simulink library "WECSim_Lib"  (R2014b)
settings: Solver=ode45  StartTime=0.0  StopTime=10.0  RelTol=1e-3
undefined symbols (not defined in the file): body, constraint, pto, simu, waves, X, Y, Z
libraries: nesl_utility x178, sm_lib x59, vrlib x12
(part 4 of 6)

== system WECSim_Lib/Body Elements/Rigid Body/Structure ==
  note: SimMechanics Model
      |
      | Body: Consists of body properties (inertia and vizualisation) defined at the CG, and a connection point at (0,0,0), the free surface.
      |
      | Forces::  Total forces calculated by WEC-Sim are applied at the Body CG. Other forces (constraints and PTOs) can be applied outside of this block, though the connection point.
      |
      | Motion Sensor: Measures the displacement, velocity, and acceleration of the Body CG relative to the world frame.
  note: body.mass
      | body.momOfInertia
      | body.geometryFile (set through Rigid Body mask)
      | body.hydroData.properties.cg
      | body.initDisp.initAngularDispAxis
      | body.initDisp.initAngularDispAngle
      | body.initDisp.initLinDisp
  Total Force : Inport
  Body Properties : sm_lib/Body Elements/Solid  InertiaType=Custom  Mass=body.mass  MassUnits=kg  CenterOfMass=[0 0 0]  CenterOfMassUnits=m  MomentsOfInertia=body.momOfInertia  MomentsOfInertiaUnits=kg*m^2  ProductsOfInertia=[0 0 0]  ProductsOfInertiaUnits=kg*m^2  DensityBased=on  Density=1000  DensityUnits=kg/(m^3)  GraphicType=FromGeometry  MarkerShape=Sphere  MarkerSize=10  MarkerSizeUnits=m  GraphicVisPropType=SimpleVisualProperties  GraphicDiffuseColor=body.viz.color  GraphicSpecularColor=[0.5 0.5 0.5 1.0]  GraphicAmbientColor=[0.15 0.15 0.15 1.0]  GraphicEmissiveColor=[0.0 0.0 0.0 1.0]  GraphicShininess=75  GraphicOpacity=body.viz.opacity  GeometryShape=FromFile  RectangleSize=[1 1]  RectangleSizeUnits=m  BrickDimensions=[1 1 1]  BrickDimensionUnits=m  CylinderRadius=1  CylinderRadiusUnits=m  CylinderLength=1  CylinderLengthUnits=m  SphereRadius=1  SphereRadiusUnits=m  EllipsoidRadii=[1 1 1]  EllipsoidRadiiUnits=m  ExtrusionCrossSection=[1 1; -1 1; -1 -1; 1 -1]  ExtrusionCrossSectionUnits=m  ExtrusionLength=1  ExtrusionLengthUnits=m  PolygonNumSides=3  PolygonOuterRadius=1  PolygonOuterRadiusUnits=m  ExtGeomFileType=STL  ExtGeomFileName=geometry/float.stl  ExtGeomFileUnits=m  RevolutionCrossSection=[1 1; 1 -1; 2 -1; 2 1]  RevolutionCrossSectionUnits=m  RevolutionExtent=Full  RevolutionAngle=180  RevolutionAngleUnits=deg  BlockFunction=simmechanics.library.body_elements.solid
  External Force and Torque : sm_lib/Forces and Torques/External Force and Torque  ForceResolutionFrame=World  EnableForceX=off  EnableForceY=off  EnableForceZ=off  EnableForce=on  TorqueResolutionFrame=World  EnableTorqueX=off  EnableTorqueY=off  EnableTorqueZ=off  EnableTorque=on  BlockFunction=simmechanics.library.forces_torques.external_force_torque
  Motion Sensor : Subsystem
  Rigid Transform (Setup CG) : sm_lib/Frames and Transforms/Rigid Transform  TranslationMethod=Cartesian  TranslationLengthUnit=m  TranslationStandardAxis=+Z  TranslationStandardOffset=0  TranslationCartesianOffset=body.hydroData.properties.cg  TranslationROffset=0  TranslationROffsetUnits=m  TranslationZOffset=0  TranslationZOffsetUnits=m  TranslationThetaOffset=0  TranslationThetaOffsetUnits=deg  RotationMethod=None  RotationAngleUnits=rad  RotationStandardAxis=+Y  RotationAngle=0.05  RotationArbitraryAxis=[0.57735026918962584 0.57735026918962584 0.57735026918962584]  FollAlignAxisA=+X  BaseAlignAxisA=+Y  FollAlignAxisB=+Y  BaseAlignAxisB=+Z  RotationMatrix=[1 0 0; 0 1 0; 0 0 1]  BlockFunction=simmechanics.library.frames_transforms.rigid_transform
  Rigid Transform (Setup Initial Disp) : sm_lib/Frames and Transforms/Rigid Transform  TranslationMethod=Cartesian  TranslationLengthUnit=m  TranslationStandardAxis=+Z  TranslationStandardOffset=0  TranslationCartesianOffset=body.initDisp.initLinDisp  TranslationROffset=0  TranslationROffsetUnits=m  TranslationZOffset=0  TranslationZOffsetUnits=m  TranslationThetaOffset=0  TranslationThetaOffsetUnits=deg  RotationMethod=ArbitraryAxis  RotationAngleUnits=rad  RotationStandardAxis=+Y  RotationAngle=body.initDisp.initAngularDispAngle  RotationArbitraryAxis=body.initDisp.initAngularDispAxis  FollAlignAxisA=+X  BaseAlignAxisA=+Y  FollAlignAxisB=+Y  BaseAlignAxisB=+Z  RotationMatrix=[1 0 0; 0 1 0; 0 0 1]  BlockFunction=simmechanics.library.frames_transforms.rigid_transform
  Selector : Selector  InputPortWidth=6  Indices=[1:3]
  Selector1 : Selector  InputPortWidth=6  Indices=[4:6]
  Simulink-PS Converter1 : nesl_utility/Simulink-PS Converter  PhysicalDomain=network_engine_domain  SubClassName=ps_input  LeftPortType=input  RightPortType=output  PseudoPeriodic=off  Frequencies=[]  NoiseDistribution=none  NoiseParameters=[]  Unit=1  AffineConversion=off  InputFiltering=off  SimscapeFilterOrder=1  InputFilterTimeConstant=0.001  UdotUserProvided=1
  Simulink-PS Converter2 : nesl_utility/Simulink-PS Converter  PhysicalDomain=network_engine_domain  SubClassName=ps_input  LeftPortType=input  RightPortType=output  PseudoPeriodic=off  Frequencies=[]  NoiseDistribution=none  NoiseParameters=[]  Unit=1  AffineConversion=off  InputFiltering=off  SimscapeFilterOrder=1  InputFilterTimeConstant=0.001  UdotUserProvided=1
  World Frame : sm_lib/Frames and Transforms/World Frame  BlockFunction=simmechanics.library.frames_transforms.world_frame
  Conn Free Surface : PMIOPort  Port=1  Side=Right
  Response : Outport
  wires:
  Motion Sensor/1(Response) -> Response/1
  Selector1/1 -> Simulink-PS Converter2/1
  Selector/1 -> Simulink-PS Converter1/1
  Total Force/1 -> Selector/1, Selector1/1
  connections:
  World Frame/RConn1 -- Motion Sensor/LConn1
  Rigid Transform (Setup Initial Disp)/LConn1 -- Rigid Transform (Setup CG)/RConn1
  Conn Free Surface/RConn1 -- Rigid Transform (Setup CG)/LConn1
  Motion Sensor/RConn1 -- External Force and Torque/RConn1 -- Body Properties/RConn1 -- Rigid Transform (Setup Initial Disp)/RConn1
  External Force and Torque/LConn2 -- Simulink-PS Converter2/RConn1
  External Force and Torque/LConn1 -- Simulink-PS Converter1/RConn1

== system WECSim_Lib/Body Elements/Rigid Body/Wave Diffraction and Excitation Force Calculation ==
  note: Calculates the excitation force, F_Excitation, given by
      | F_Excitation = R * F_wave.
      |
      | There are two cases for Calculating the Ramp function, R:
      |    1. simulation Time is less than Ramp Time: Apply ramp function
      |    2. Simulation time is larger than Ramp Time: Do not apply ramp function (R=1)
      |
      | Similarly there are two cases for the wave force, F_wave: Regular and Irregular waves.
      |
      | Notes:
      | Output dimension set to '6' in output port to eliminate singleton dimension.
  Time : Inport
  Displacement : Inport  Port=2
  WaveElv : Inport  Port=3
  Add : Sum
  If2 : If  NumInputs=2  IfExpression=u1 < u2
  Linear Wave Excitation Force Variant Subsystem : Subsystem  Variant=on
  Merge1 : Merge
  No Ramp Function : Subsystem  TreatAsAtomicUnit=on
  Nonlinear FK Force Variant Subsystem : Subsystem  Variant=on
  Product : Product
  Ramp Function : Subsystem  TreatAsAtomicUnit=on
  Ramp Function Time1 : Constant  Value=simu.rampT
  F_Excitation : Outport  PortDimensions=6
  wires:
  No Ramp Function/1(R) -> Merge1/2
  Ramp Function/1(R) -> Merge1/1
  If2/1 -> Ramp Function/Action
  If2/2 -> No Ramp Function/Action
  Ramp Function Time1/1 -> If2/2
  Merge1/1 -> Product/1  "R"
  Time/1 -> Linear Wave Excitation Force Variant Subsystem/1(In1), Nonlinear FK Force Variant Subsystem/1(In1), Ramp Function/1(Time), If2/1
  Add/1 -> Product/2  "F_wave"
  Product/1 -> F_Excitation/1  "F_Excitation"
  Displacement/1 -> Nonlinear FK Force Variant Subsystem/2(In2)
  WaveElv/1 -> Nonlinear FK Force Variant Subsystem/3(In3)
  Linear Wave Excitation Force Variant Subsystem/1(Out1) -> Add/1
  Nonlinear FK Force Variant Subsystem/1(Out1) -> Add/2

== system WECSim_Lib/Body Elements/Rigid Body/Wave Radiation Forces Calculation ==
  note: Calculates the wave radiation forces:
      | 	Added Mass Force = added mass matrix * acceleration vector
      | 	Single frequency radiation damping force = radiation damping matrix * acceleration vector
      | 	Convolution Integral
      |
      | The code can run in one of two modes:
      | 	Convolution integral: the radiation damping matrix is set to zero, and the infinite frequency added mass is used.
      | 	Single Frequency: The impulse response function K is set to zero, and the radiation damping and added mass matrices for the specified frequency are used.
      |
      | This is set by the body.hydroForcePre method, based on the specified wave type.
  Velocity : Inport
  Acceleration : Inport  Port=2
  Time : Inport  Port=3
  Added Mass Matrix : Constant  Value=body.hydroForce.fAddedMass
  Product1 : Product  Multiplication=Matrix(*)
  SS CI and Constant-Damping-CoeVariant Subsystem : Subsystem  Variant=on
  Transport Delay : TransportDelay  DelayTime=10e-8
  F_RadiationDamping : Outport
  F_AddedMass : Outport  Port=2
  wires:
  Added Mass Matrix/1 -> Product1/1
  Product1/1 -> F_AddedMass/1  "F_AddedMass"
  Velocity/1 -> SS CI and Constant-Damping-CoeVariant Subsystem/1(In1)
  SS CI and Constant-Damping-CoeVariant Subsystem/1(Out1) -> F_RadiationDamping/1  "F_RadiationDamping"
  Transport Delay/1 -> Product1/2
  Acceleration/1 -> Transport Delay/1
  Time/1 -> SS CI and Constant-Damping-CoeVariant Subsystem/2(In2)

== system WECSim_Lib/Constraints/Floating (3DOF)/Mooring ==
  note: 1) Add Subsystem or Model blocks as valid variant choices.
      | 2) You cannot connect blocks at this level. At simulation, connectivity is automatically
      | determined, based on the active variant and port name matching.
  Displacement : Inport
  Clock : Inport  Port=2
  Velocity : Inport  Port=3
  MoorDyn : Subsystem  VariantControl=sv_moorDyn
  Mooring Matrix : Subsystem  VariantControl=sv_mooringMatrix
  F_Mooring : Outport

== system WECSim_Lib/Constraints/Floating (6DOF)/Mooring ==
  note: 1) Add Subsystem or Model blocks as valid variant choices.
      | 2) You cannot connect blocks at this level. At simulation, connectivity is automatically
      | determined, based on the active variant and port name matching.
  Displacement : Inport
  Clock : Inport  Port=2
  Velocity : Inport  Port=3
  MoorDyn : Subsystem  VariantControl=sv_moorDyn
  Mooring Matrix : Subsystem  VariantControl=sv_mooringMatrix
  F_Mooring : Outport

== system WECSim_Lib/Constraints/Heave/Mooring ==
  note: 1) Add Subsystem or Model blocks as valid variant choices.
      | 2) You cannot connect blocks at this level. At simulation, connectivity is automatically
      | determined, based on the active variant and port name matching.
  Displacement : Inport
  Clock : Inport  Port=2
  Velocity : Inport  Port=3
  MoorDyn : Subsystem  VariantControl=sv_moorDyn
  Mooring Matrix : Subsystem  VariantControl=sv_mooringMatrix
  F_Mooring : Outport

== system WECSim_Lib/Constraints/Pitch/Mooring ==
  note: 1) Add Subsystem or Model blocks as valid variant choices.
      | 2) You cannot connect blocks at this level. At simulation, connectivity is automatically
      | determined, based on the active variant and port name matching.
  Displacement : Inport
  Clock : Inport  Port=2
  Velocity : Inport  Port=3
  MoorDyn : Subsystem  VariantControl=sv_moorDyn
  Mooring Matrix : Subsystem  VariantControl=sv_mooringMatrix
  F_Mooring : Outport

== system WECSim_Lib/Constraints/Surge/Mooring ==
  note: 1) Add Subsystem or Model blocks as valid variant choices.
      | 2) You cannot connect blocks at this level. At simulation, connectivity is automatically
      | determined, based on the active variant and port name matching.
  Displacement : Inport
  Clock : Inport  Port=2
  Velocity : Inport  Port=3
  MoorDyn : Subsystem  VariantControl=sv_moorDyn
  Mooring Matrix : Subsystem  VariantControl=sv_mooringMatrix
  F_Mooring : Outport

== system WECSim_Lib/PTOs/Rotational PTO (Local RY)/InternalMechanics ==
  note: Calculate PTO force and power.
      |
      | F_pto  = k*x + c*v,
      | where F_pto is the force the PTO applies to the body (at the PTO location), x and v are the joint position and velocity.
      |
      | The power extracted is
      | P = c * v^2
  Position : Inport
  Velocity : Inport  Port=2
  Add : Sum  Inputs=--
  Math Function : Math  Operator=square  SaturateOnIntegerOverflow=on
  PCC Damping Coefficient : Constant  Value=pto.c
  PCC Stiffness Coefficient : Constant  Value=pto.k
  Product : Product  Inputs=**
  Product1 : Product  Inputs=**
  Product2 : Product  Inputs=**
  Force : Outport
  Power : Outport  Port=2
  wires:
  PCC Damping Coefficient/1 -> Product2/1, Product1/1
  Product2/1 -> Power/1
  Velocity/1 -> Math Function/1, Product1/2
  PCC Stiffness Coefficient/1 -> Product/2
  Position/1 -> Product/1
  Add/1 -> Force/1
  Math Function/1 -> Product2/2
  Product/1 -> Add/1
  Product1/1 -> Add/2

== system WECSim_Lib/PTOs/Rotational PTO Prescribed Motion (Local RY)/InternalMechanics ==
  note: Calculate PTO force and power.
      |
      | F_pto  = k*x + c*v,
      | where F_pto is the force the PTO applies to the body (at the PTO location), x and v are the joint position and velocity.
      |
      | The power extracted is
      | P = c * v^2
  Position : Inport
  Velocity : Inport  Port=2
  Add : Sum  Inputs=--
  Math Function : Math  Operator=square  SaturateOnIntegerOverflow=on
  PCC Damping Coefficient : Constant  Value=pto.c
  PCC Stiffness Coefficient : Constant  Value=pto.k
  Product : Product  Inputs=**
  Product1 : Product  Inputs=**
  Product2 : Product  Inputs=**
  Force : Outport
  Power : Outport  Port=2
  wires:
  PCC Damping Coefficient/1 -> Product2/1, Product1/1
  Product2/1 -> Power/1
  Velocity/1 -> Math Function/1, Product1/2
  PCC Stiffness Coefficient/1 -> Product/2
  Position/1 -> Product/1
  Add/1 -> Force/1
  Math Function/1 -> Product2/2
  Product/1 -> Add/1
  Product1/1 -> Add/2

== system WECSim_Lib/PTOs/Rotational PTO UD Torque (Local RY)/InternalMechanics ==
  note: Calculate PTO force and power.
      |
      | F_pto  = k*x + c*v,
      | where F_pto is the force the PTO applies to the body (at the PTO location), x and v are the joint position and velocity.
      |
      | The power extracted is
      | P = c * v^2
  Position : Inport
  Velocity : Inport  Port=2
  Add : Sum  Inputs=--
  Math Function : Math  Operator=square  SaturateOnIntegerOverflow=on
  PCC Damping Coefficient : Constant  Value=pto.c
  PCC Stiffness Coefficient : Constant  Value=pto.k
  Product : Product  Inputs=**
  Product1 : Product  Inputs=**
  Product2 : Product  Inputs=**
  Force : Outport
  Power : Outport  Port=2
  wires:
  Product1/1 -> Add/2
  Product/1 -> Add/1
  Math Function/1 -> Product2/2
  Add/1 -> Force/1
  Position/1 -> Product/1
  PCC Stiffness Coefficient/1 -> Product/2
  Velocity/1 -> Product1/2, Math Function/1
  Product2/1 -> Power/1
  PCC Damping Coefficient/1 -> Product1/1, Product2/1

== system WECSim_Lib/PTOs/Translational PTO (Local X)/ForceAndPower ==
  note: Calculate PTO force and power.
      |
      | F_pto  = k*x + c*v,
      | where F_pto is the force the PTO applies to the body (at the PTO location), x and v are the joint position and velocity.
      |
      | The power extracted is
      | P = c * v^2
  Pos : Inport
  Vel : Inport  Port=2
  Add : Sum  Inputs=--
  Math Function : Math  Operator=square  SaturateOnIntegerOverflow=on
  PCC Damping Coefficient : Constant  Value=pto.c
  PCC Stiffness Coefficient : Constant  Value=pto.k
  Product : Product  Inputs=**
  Product1 : Product  Inputs=**
  Product2 : Product  Inputs=**
  Force : Outport
  Power : Outport  Port=2
  wires:
  PCC Damping Coefficient/1 -> Product1/1, Product2/1
  Product2/1 -> Power/1
  Vel/1 -> Product1/2, Math Function/1
  PCC Stiffness Coefficient/1 -> Product/2
  Pos/1 -> Product/1
  Add/1 -> Force/1
  Math Function/1 -> Product2/2
  Product/1 -> Add/1
  Product1/1 -> Add/2

== system WECSim_Lib/PTOs/Translational PTO (Local Z)/InternalMechanics ==
  note: Calculate PTO force and power.
      |
      | F_pto  = k*x + c*v,
      | where F_pto is the force the PTO applies to the body (at the PTO location), x and v are the joint position and velocity.
      |
      | The power extracted is
      | P = c * v^2
  Position : Inport
  Velocity : Inport  Port=2
  Add : Sum  Inputs=--
  Math Function : Math  Operator=square  SaturateOnIntegerOverflow=on
  PCC Damping Coefficient : Constant  Value=pto.c
  PCC Stiffness Coefficient : Constant  Value=pto.k
  Product : Product  Inputs=**
  Product1 : Product  Inputs=**
  Product2 : Product  Inputs=**
  Force : Outport
  Power : Outport  Port=2
  wires:
  PCC Damping Coefficient/1 -> Product2/1, Product1/1
  Product2/1 -> Power/1
  Velocity/1 -> Math Function/1, Product1/2
  PCC Stiffness Coefficient/1 -> Product/2
  Position/1 -> Product/1
  Add/1 -> Force/1
  Math Function/1 -> Product2/2
  Product/1 -> Add/1
  Product1/1 -> Add/2

== system WECSim_Lib/PTOs/Translational PTO Prescribed Motion (Local X)/ForceAndPower ==
  note: Calculate PTO force and power.
      |
      | F_pto  = k*x + c*v,
      | where F_pto is the force the PTO applies to the body (at the PTO location), x and v are the joint position and velocity.
      |
      | The power extracted is
      | P = c * v^2
  Pos : Inport
  Vel : Inport  Port=2
  Add : Sum  Inputs=--
  Math Function : Math  Operator=square  SaturateOnIntegerOverflow=on
  PCC Damping Coefficient : Constant  Value=pto.c
  PCC Stiffness Coefficient : Constant  Value=pto.k
  Product : Product  Inputs=**
  Product1 : Product  Inputs=**
  Product2 : Product  Inputs=**
  Force : Outport
  Power : Outport  Port=2
  wires:
  Product1/1 -> Add/2
  Product/1 -> Add/1
  Math Function/1 -> Product2/2
  Add/1 -> Force/1
  Pos/1 -> Product/1
  PCC Stiffness Coefficient/1 -> Product/2
  Vel/1 -> Math Function/1, Product1/2
  Product2/1 -> Power/1
  PCC Damping Coefficient/1 -> Product2/1, Product1/1

== system WECSim_Lib/PTOs/Translational PTO Prescribed Motion (Local Z)/InternalMechanics ==
  note: Calculate PTO force and power.
      |
      | F_pto  = k*x + c*v,
      | where F_pto is the force the PTO applies to the body (at the PTO location), x and v are the joint position and velocity.
      |
      | The power extracted is
      | P = c * v^2
  Position : Inport
  Velocity : Inport  Port=2
  Add : Sum  Inputs=--
  Math Function : Math  Operator=square  SaturateOnIntegerOverflow=on
  PCC Damping Coefficient : Constant  Value=pto.c
  PCC Stiffness Coefficient : Constant  Value=pto.k
  Product : Product  Inputs=**
  Product1 : Product  Inputs=**
  Product2 : Product  Inputs=**
  Force : Outport
  Power : Outport  Port=2
  wires:
  PCC Damping Coefficient/1 -> Product2/1, Product1/1
  Product2/1 -> Power/1
  Velocity/1 -> Math Function/1, Product1/2
  PCC Stiffness Coefficient/1 -> Product/2
  Position/1 -> Product/1
  Add/1 -> Force/1
  Math Function/1 -> Product2/2
  Product/1 -> Add/1
  Product1/1 -> Add/2

== system WECSim_Lib/PTOs/Translational PTO UD Force (Local X)/ForceAndPower ==
  note: Calculate PTO force and power.
      |
      | F_pto  = k*x + c*v,
      | where F_pto is the force the PTO applies to the body (at the PTO location), x and v are the joint position and velocity.
      |
      | The power extracted is
      | P = c * v^2
  Pos : Inport
  Vel : Inport  Port=2
  Add : Sum  Inputs=--
  Math Function : Math  Operator=square  SaturateOnIntegerOverflow=on
  PCC Damping Coefficient : Constant  Value=pto.c
  PCC Stiffness Coefficient : Constant  Value=pto.k
  Product : Product  Inputs=**
  Product1 : Product  Inputs=**
  Product2 : Product  Inputs=**
  Force : Outport
  Power : Outport  Port=2
  wires:
  PCC Damping Coefficient/1 -> Product1/1, Product2/1
  Product2/1 -> Power/1
  Vel/1 -> Product1/2, Math Function/1
  PCC Stiffness Coefficient/1 -> Product/2
  Pos/1 -> Product/1
  Add/1 -> Force/1
  Math Function/1 -> Product2/2
  Product/1 -> Add/1
  Product1/1 -> Add/2

== system WECSim_Lib/PTOs/Translational PTO UD Force (Local Z)/InternalMechanics ==
  note: Calculate PTO force and power.
      |
      | F_pto  = k*x + c*v,
      | where F_pto is the force the PTO applies to the body (at the PTO location), x and v are the joint position and velocity.
      |
      | The power extracted is
      | P = c * v^2
  Position : Inport
  Velocity : Inport  Port=2
  Add : Sum  Inputs=--
  Math Function : Math  Operator=square  SaturateOnIntegerOverflow=on
  PCC Damping Coefficient : Constant  Value=pto.c
  PCC Stiffness Coefficient : Constant  Value=pto.k
  Product : Product  Inputs=**
  Product1 : Product  Inputs=**
  Product2 : Product  Inputs=**
  Force : Outport
  Power : Outport  Port=2
  wires:
  Product1/1 -> Add/2
  Product/1 -> Add/1
  Math Function/1 -> Product2/2
  Add/1 -> Force/1
  Position/1 -> Product/1
  PCC Stiffness Coefficient/1 -> Product/2
  Velocity/1 -> Product1/2, Math Function/1
  Product2/1 -> Power/1
  PCC Damping Coefficient/1 -> Product1/1, Product2/1

== system WECSim_Lib/Body Elements/Rigid Body/B2B Subsystem/B2B ==
  CrossCoupling : Subsystem  mask{body=body}
      mask prompts: body "Body Number"
      mask help: This is used to
      mask init:
      | %In the initialization tab we place the code modifying the block
      | 
      | cb = gcb;
      | % position of initial blocks
      | set_param([cb '/vel1'],'Position',[200 1*50 240 (1*50+30)])
      | set_param([cb '/BC1'], 'Position',[375 40 380 90])
      | set_param([cb '/vel'], 'Position',[410 59 440 71])
      | set_param([cb '/acc1'],'Position',[600 1*50 640 (1*50+30)])
      | set_param([cb '/BC2'], 'Position',[775 40 780 90])
      | set_param([cb '/acc'], 'Position',[810 59 840 71])
      | 
      | % add/delete lines & blocks
      | newInputs = 0;
      | numbodies = body.bodyTotal;
      | iBod = 2;
      | while iBod < 100
      |     try 
      |         find_system([cb,'/vel',num2str(iBod)],'Type','Block');
      |         if iBod > numbodies
      |             %delete 'From' blocks and lines if bodynumber > total bodies
      |             delete_line(cb,['vel',num2str(iBod),'/1'],['BC',num2str(1),'/',num2str(iBod)])
      |             delete_line(cb,['acc',num2str(iBod),'/1'],['BC',num2str(2),'/',num2str(iBod)])
      |             delete_block([cb '/vel',num2str(iBod)])
      |             delete_block([cb '/acc',num2str(iBod)])
      |         end
      |     catch
      |         %set number of outputs for 'Bus Creator' blocks 
      |         if newInputs==0
      |             set_param([cb,'/BC1'],'Inputs',num2str(numbodies))
      |             set_param([cb,'/BC2'],'Inputs',num2str(numbodies))
      |         end
      |         if iBod <= numbodies
      |             newInputs = newInputs + 1;
      |             %add velocity 'From' block
      |             add_block('simulink/Signal Routing/From', [cb,'/vel',num2str(iBod)],'MakeNameUnique', 'on',...
      |             'Position',[200 iBod*50 240 (iBod*50+30)], 'BackgroundColor','green')
      |             h=[cb,'/vel',num2str(iBod)];
      |             responseName=['vel' num2str(iBod)];
      |             set_param(h,'GotoTag',responseName);
      |             %add acceleration 'From' block
      |             add_block('simulink/Signal Routing/From', [cb,'/acc',num2str(iBod)],'MakeNameUnique', 'on',...
      |             'Position',[600 iBod*50 640 (iBod*50+30)], 'BackgroundColor','green')
      |             h=[cb,'/acc',num2str(iBod)];
      |             responseName=['acc' num2str(iBod)];
      |             set_param(h,'GotoTag',responseName);
      |             %add lines
      |             add_line(cb,['vel',num2str(iBod),'/1'],['BC',num2str(1),'/',num2str(iBod)])
      |             add_line(cb,['acc',num2str(iBod),'/1'],['BC',num2str(2),'/',num2str(iBod)])
      |         else
      |             break
      |         end
      |     end
      |     iBod = iBod + 1;
      | end
      mask Callback body: %customsat_callback('input',gcb)
      mask DialogControl DescTextVar Prompt: This block transfers the velocity and acceleration vectors between bodies allowing for the coupled hydrodynamic forces to be calculated.  This block should not be included if there is only one body or if the hydrodynamic coupling parameter is set to 'No' in the rigid body block.
  vel : Outport
  acc : Outport  Port=2
  wires:
  CrossCoupling/1(vel) -> vel/1
  CrossCoupling/2(acc) -> acc/1

== system WECSim_Lib/Body Elements/Rigid Body/B2B Subsystem/noB2B ==
  vel_in : Inport
  acc_in : Inport  Port=2
  vel : Outport
  acc : Outport  Port=2
  wires:
  vel_in/1 -> vel/1  "x"
  acc_in/1 -> acc/1

== system WECSim_Lib/Body Elements/Rigid Body/Hydrostatic Restoring Force Calculation/Linear and Nonlinear Restoring Force Variant Subsystem ==
  note: 1) Add Subsystem or Model blocks as valid variant choices.
      | 2) You cannot connect blocks at this level. At simulation, connectivity is automatically
      | determined, based on the active variant and port name matching.
  In1 : Inport
  In2 : Inport  Port=2
  In3 : Inport  Port=3
  "Linear Hydrostatic Restoring Force " : Subsystem  VariantControl=sv_linearHydro
  Nonlinear Hydrostatic Restoring Force : Subsystem  VariantControl=sv_nonlinearHydro
  Out1 : Outport

== system WECSim_Lib/Body Elements/Rigid Body/Morrison Element and ViscousDampingForceCalculation/Morrison Element Variant Subsystem ==
  note: 1) Add Subsystem or Model blocks as valid variant choices.
      | 2) You cannot connect blocks at this level. At simulation, connectivity is automatically
      | determined, based on the active variant and port name matching.
  In1 : Inport
  In2 : Inport  Port=2
  In3 : Inport  Port=3
  Morrison Element Off : Subsystem  VariantControl=sv_MEOff
  Morrison Element On : Subsystem  Variant=on  VariantControl=sv_MEOn
  Out1 : Outport

== system WECSim_Lib/Body Elements/Rigid Body/Nonlinear Wave Elevation/Linear or Instantaneous Free Surface ==
  note: 1) Add Subsystem or Model blocks as valid variant choices.
      | 2) You cannot connect blocks at this level. At simulation, connectivity is automatically
      | determined, based on the active variant and port name matching.
  In1 : Inport
  In2 : Inport  Port=2
  "Instantaneous Water Free Surface  " : Subsystem  VariantControl=sv_instFS
  "Mean Water Free Surface " : Subsystem  VariantControl=sv_meanFS
  Out1 : Outport

== system WECSim_Lib/Body Elements/Rigid Body/Structure/Motion Sensor ==
  note: Measures the position, velocity, and acceleration of the follower (F) frame relative to the base (B) frame.
      | Ouputs a bus of 3 signals, each signal is a vector length 6.
  Angle : MATLAB Function  TreatAsAtomicUnit=on
  Bus Creator : BusCreator  Inputs=3
  Mux : Mux
  Mux1 : Mux  Inputs=6
  Mux2 : Mux  Inputs=6
  PS-Simulink Converter{,1..15} (16 alike) : nesl_utility/PS-Simulink Converter  PhysicalDomain=network_engine_domain  SubClassName=ps_output  LeftPortType=input  RightPortType=output  PseudoPeriodic=off  Frequencies=[]  Unit=1  AffineConversion=off
  Transform Sensor : sm_lib/Frames and Transforms/Transform Sensor  MeasurementFrame=World  SenseAngle=off  SenseAxis=off  SenseAngle1=off  SenseAngle2=off  SenseAngle3=off  SenseQ=on  SenseR=off  SenseOmegaX=on  SenseOmegaY=on  SenseOmegaZ=on  SenseOmega1=off  SenseOmega2=off  SenseOmega3=off  SenseQDot=off  SenseRDot=off  SenseAlphaX=on  SenseAlphaY=on  SenseAlphaZ=on  SenseAlpha1=off  SenseAlpha2=off  SenseAlpha3=off  SenseQDDot=off  SenseRDDot=off  SenseX=on  SenseY=on  SenseZ=on  SenseRad=off  SenseAzim=off  SenseDist=off  SenseInc=off  SenseXDot=on  SenseYDot=on  SenseZDot=on  SenseRadDot=off  SenseAzimDot=off  SenseDistDot=off  SenseIncDot=off  SenseXDDot=on  SenseYDDot=on  SenseZDDot=on  SenseRadDDot=off  SenseAzimDDot=off  SenseDistDDot=off  SenseIncDDot=off  BlockFunction=simmechanics.library.frames_transforms.transform_sensor
  F : PMIOPort  Port=1  Side=Right
  B : PMIOPort  Port=2  Side=Left
  Response : Outport
  wires:
  Bus Creator/1 -> Response/1
  PS-Simulink Converter15/1 -> Mux2/3  "az"
  PS-Simulink Converter3/1 -> Mux1/6  "omegaz"
  PS-Simulink Converter11/1 -> Mux1/2  "vy"
  PS-Simulink Converter2/1 -> Mux1/5  "omegay"
  PS-Simulink Converter1/1 -> Mux1/4  "omegax"
  PS-Simulink Converter6/1 -> Mux2/6  "alphaz"
  PS-Simulink Converter5/1 -> Mux2/5  "alphay"
  PS-Simulink Converter9/1 -> Mux/3  "z"
  PS-Simulink Converter8/1 -> Mux/2  "y"
  PS-Simulink Converter7/1 -> Mux/1  "x"
  Angle/1(E) -> Mux/4
  Mux2/1 -> Bus Creator/3  "acc"
  Mux1/1 -> Bus Creator/2  "vel"
  Mux/1 -> Bus Creator/1  "disp"
  PS-Simulink Converter14/1 -> Mux2/2  "ay"
  PS-Simulink Converter13/1 -> Mux2/1  "ax"
  PS-Simulink Converter12/1 -> Mux1/3  "vz"
  PS-Simulink Converter10/1 -> Mux1/1  "vx"
  PS-Simulink Converter4/1 -> Mux2/4  "alphax"
  PS-Simulink Converter/1 -> Angle/1(Q)
  connections:
  PS-Simulink Converter3/LConn1 -- Transform Sensor/RConn5
  PS-Simulink Converter2/LConn1 -- Transform Sensor/RConn4
  PS-Simulink Converter1/LConn1 -- Transform Sensor/RConn3
  PS-Simulink Converter6/LConn1 -- Transform Sensor/RConn8
  PS-Simulink Converter5/LConn1 -- Transform Sensor/RConn7
  PS-Simulink Converter4/LConn1 -- Transform Sensor/RConn6
  PS-Simulink Converter7/LConn1 -- Transform Sensor/RConn9
  PS-Simulink Converter8/LConn1 -- Transform Sensor/RConn10
  PS-Simulink Converter9/LConn1 -- Transform Sensor/RConn11
  PS-Simulink Converter10/LConn1 -- Transform Sensor/RConn12
  PS-Simulink Converter11/LConn1 -- Transform Sensor/RConn13
  PS-Simulink Converter12/LConn1 -- Transform Sensor/RConn14
  PS-Simulink Converter13/LConn1 -- Transform Sensor/RConn15
  PS-Simulink Converter14/LConn1 -- Transform Sensor/RConn16
  PS-Simulink Converter15/LConn1 -- Transform Sensor/RConn17
  Transform Sensor/RConn2 -- PS-Simulink Converter/LConn1
  B/RConn1 -- Transform Sensor/LConn1
  Transform Sensor/RConn1 -- F/RConn1

== system WECSim_Lib/Body Elements/Rigid Body/Wave Diffraction and Excitation Force Calculation/Linear Wave Excitation Force Variant Subsystem ==
  note: 1) Add Subsystem or Model blocks as valid variant choices.
      | 2) You cannot connect blocks at this level. At simulation, connectivity is automatically
      | determined, based on the active variant and port name matching.
  In1 : Inport
  Irregular Wave Excitation Force : Subsystem  VariantControl=sv_irregularWaves
  No Wave Excitation Force : Subsystem  VariantControl=sv_noWave
  Regular Wave Excitation Force : Subsystem  VariantControl=sv_regularWaves
  User Defined Wave Excitation Force : Subsystem  VariantControl=sv_udfWaves
  Out1 : Outport

== system WECSim_Lib/Body Elements/Rigid Body/Wave Diffraction and Excitation Force Calculation/No Ramp Function ==
  note: No ramp function applied.
      | R = 1
      |
      | Note:
      | Output port initial value also set to 1,
  Action Port : ActionPort
  Constant : Constant
  R : Outport  InitialOutput=1
  wires:
  Constant/1 -> R/1

== system WECSim_Lib/Body Elements/Rigid Body/Wave Diffraction and Excitation Force Calculation/Nonlinear FK Force Variant Subsystem ==
  note: 1) Add Subsystem or Model blocks as valid variant choices.
      | 2) You cannot connect blocks at this level. At simulation, connectivity is automatically
      | determined, based on the active variant and port name matching.
  In1 : Inport
  In2 : Inport  Port=2
  In3 : Inport  Port=3
  No Nonlinear FroudeKrylov Force : Subsystem  VariantControl=sv_linearHydro
  With Nonlinear FroudeKrylov Force : Subsystem  VariantControl=sv_nonlinearHydro
  Out1 : Outport

== system WECSim_Lib/Body Elements/Rigid Body/Wave Diffraction and Excitation Force Calculation/Ramp Function ==
  note: Calculates the ramp function, R, given by
      |
      | R = (1 / 2)  * (1 + sin( (pi / t_ramp) * t  +  ((3 / 2) * pi) ) ).
  Time : Inport
  Action Port : ActionPort
  Add : Sum
  Add1 : Sum
  Constant : Constant  Value=1/2
  Constant1 : Constant
  Constant2 : Constant  Value=3*pi/2
  Constant3 : Constant  Value=pi
  Divide : Product  Inputs=*/
  Product : Product
  Product1 : Product
  Ramp Time : Constant  Value=simu.rampT
  Sine Wave Function : Sin  TimeSource=Use external signal  SampleTime=0
  R : Outport
  wires:
  Add/1 -> Product/1
  Sine Wave Function/1 -> Add/2
  Constant1/1 -> Add/1
  Constant/1 -> Product/2
  Product/1 -> R/1
  Time/1 -> Product1/1  "t"
  Ramp Time/1 -> Divide/2  "t_ramp"
  Constant2/1 -> Add1/2  "phase"
  Add1/1 -> Sine Wave Function/1
  Product1/1 -> Add1/1
  Constant3/1 -> Divide/1
  Divide/1 -> Product1/2  "frequency"

== system WECSim_Lib/Body Elements/Rigid Body/Wave Radiation Forces Calculation/SS CI and Constant-Damping-CoeVariant Subsystem ==
  note: 1) Add Subsystem or Model blocks as valid variant choices.
      | 2) You cannot connect blocks at this level. At simulation, connectivity is automatically
      | determined, based on the active variant and port name matching.
  In1 : Inport
  In2 : Inport  Port=2
  Constant Coefficients : Subsystem  VariantControl=sv_constantCoeff
  Convolution Integral Calculation : Subsystem  VariantControl=sv_convolution
  "State-Space Calculation " : Subsystem  VariantControl=sv_stateSpace
  Out1 : Outport

== system WECSim_Lib/Constraints/Floating (3DOF)/Mooring/MoorDyn ==
  Displacement : Inport
  Clock : Inport  Port=2
  Velocity : Inport  Port=3
  MoorDyn : Subsystem  InitFcn=|  StopFcn=|
      InitFcn=|
      | % Initialize MoorDyn Lib (Windows:dll or OSX:dylib)
      | if ismac
      |     loadlibrary('Lines.dylib','MoorDyn.h');
      | else
      |    if ispc
      |       loadlibrary('Lines.dll','MoorDyn.h');
      |    else
      |       disp('Cannot run MoorDyn in this platform');
      |    end
      | end
      | calllib('Lines','LinesInit',constraint.loc,[0 0 0 0 0 0]);
      StopFcn=|
      | calllib('Lines','LinesClose');
      | unloadlibrary Lines;
      settings: CloseFcn=|
      | calllib('Lines','LinesClose');
      | unloadlibrary Lines;
  F_Mooring : Outport
  wires:
  Velocity/1 -> MoorDyn/1(Velocity)
  Displacement/1 -> MoorDyn/3(Displacement)
  Clock/1 -> MoorDyn/2(Clock)
  MoorDyn/1(Flines) -> F_Mooring/1

== system WECSim_Lib/Constraints/Floating (3DOF)/Mooring/Mooring Matrix ==
  note: Calculates the Mooring Force
      |
      | Mooring force = Kmooring matrix * displacement vector (relative to cg)
      | 	+ Cmooring matrix * velocity vector
      | 	- PreTension vector
      | F_Mooring = x_cg * Km  +  v * Cm  -  T
  Displacement : Inport
  Velocity : Inport  Port=2
  Center of Gravity2 : Constant  Value=constraint.mooring.c
  Mooring K Matrix : Constant  Value=constraint.mooring.k
  Mooring Pre-Tension : Constant  Value=constraint.mooring.preTension
  Product : Product  Multiplication=Matrix(*)
  Product1 : Product  Multiplication=Matrix(*)
  sum : Sum  Inputs=--+
  F_Mooring : Outport
  wires:
  Product/1 -> sum/1  "Km*x_cg"
  Product1/1 -> sum/2  "Cm*v"
  sum/1 -> F_Mooring/1  "F_Mooring"
  Mooring Pre-Tension/1 -> sum/3  "T"
  Displacement/1 -> Product/2  "x"
  Mooring K Matrix/1 -> Product/1  "Km"
  Velocity/1 -> Product1/2  "v"
  Center of Gravity2/1 -> Product1/1  "Cm"

== system WECSim_Lib/Constraints/Floating (6DOF)/Mooring/MoorDyn ==
  Displacement : Inport
  Clock : Inport  Port=2
  Velocity : Inport  Port=3
  MoorDyn : Subsystem  InitFcn=|  StopFcn=|
      InitFcn=|
      | % Initialize MoorDyn Lib (Windows:dll or OSX:dylib)
      | if ismac
      |     loadlibrary('Lines.dylib','MoorDyn.h');
      | else
      |    if ispc
      |       loadlibrary('Lines.dll','MoorDyn.h');
      |    else
      |       disp('Cannot run MoorDyn in this platform');
      |    end
      | end
      | calllib('Lines','LinesInit',constraint.loc,[0 0 0 0 0 0]);
      StopFcn=|
      | calllib('Lines','LinesClose');
      | unloadlibrary Lines;
      settings: CloseFcn=|
      | calllib('Lines','LinesClose');
      | unloadlibrary Lines;
  F_Mooring : Outport
  wires:
  Velocity/1 -> MoorDyn/1(Velocity)
  Displacement/1 -> MoorDyn/3(Displacement)
  Clock/1 -> MoorDyn/2(Clock)
  MoorDyn/1(Flines) -> F_Mooring/1

== system WECSim_Lib/Constraints/Floating (6DOF)/Mooring/Mooring Matrix ==
  note: Calculates the Mooring Force
      |
      | Mooring force = Kmooring matrix * displacement vector (relative to cg)
      | 	+ Cmooring matrix * velocity vector
      | 	- PreTension vector
      | F_Mooring = x_cg * Km  +  v * Cm  -  T
  Displacement : Inport
  Velocity : Inport  Port=2
  Center of Gravity2 : Constant  Value=constraint.mooring.c
  Mooring K Matrix : Constant  Value=constraint.mooring.k
  Mooring Pre-Tension : Constant  Value=constraint.mooring.preTension
  Product : Product  Multiplication=Matrix(*)
  Product1 : Product  Multiplication=Matrix(*)
  sum : Sum  Inputs=--+
  F_Mooring : Outport
  wires:
  Product/1 -> sum/1  "Km*x_cg"
  Product1/1 -> sum/2  "Cm*v"
  sum/1 -> F_Mooring/1  "F_Mooring"
  Mooring Pre-Tension/1 -> sum/3  "T"
  Displacement/1 -> Product/2  "x"
  Mooring K Matrix/1 -> Product/1  "Km"
  Velocity/1 -> Product1/2  "v"
  Center of Gravity2/1 -> Product1/1  "Cm"

== system WECSim_Lib/Constraints/Heave/Mooring/MoorDyn ==
  Displacement : Inport
  Clock : Inport  Port=2
  Velocity : Inport  Port=3
  MoorDyn : Subsystem  InitFcn=|  StopFcn=|
      InitFcn=|
      | % Initialize MoorDyn Lib (Windows:dll or OSX:dylib)
      | if ismac
      |     loadlibrary('Lines.dylib','MoorDyn.h');
      | else
      |    if ispc
      |       loadlibrary('Lines.dll','MoorDyn.h');
      |    else
      |       disp('Cannot run MoorDyn in this platform');
      |    end
      | end
      | calllib('Lines','LinesInit',constraint.loc,[0 0 0 0 0 0]);
      StopFcn=|
      | calllib('Lines','LinesClose');
      | unloadlibrary Lines;
      settings: CloseFcn=|
      | calllib('Lines','LinesClose');
      | unloadlibrary Lines;
  F_Mooring : Outport
  wires:
  MoorDyn/1(Flines) -> F_Mooring/1
  Clock/1 -> MoorDyn/2(Clock)
  Displacement/1 -> MoorDyn/3(Displacement)
  Velocity/1 -> MoorDyn/1(Velocity)

== system WECSim_Lib/Constraints/Heave/Mooring/Mooring Matrix ==
  note: Calculates the Mooring Force
      |
      | Mooring force = Kmooring matrix * displacement vector (relative to cg)
      | 	+ Cmooring matrix * velocity vector
      | 	- PreTension vector
      | F_Mooring = x_cg * Km  +  v * Cm  -  T
  Displacement : Inport
  Velocity : Inport  Port=2
  Center of Gravity2 : Constant  Value=constraint.mooring.c
  Mooring K Matrix : Constant  Value=constraint.mooring.k
  Mooring Pre-Tension : Constant  Value=constraint.mooring.preTension
  Product : Product  Multiplication=Matrix(*)
  Product1 : Product  Multiplication=Matrix(*)
  sum : Sum  Inputs=--+
  F_Mooring : Outport
  wires:
  Center of Gravity2/1 -> Product1/1  "Cm"
  Velocity/1 -> Product1/2  "v"
  Mooring K Matrix/1 -> Product/1  "Km"
  Displacement/1 -> Product/2  "x"
  Mooring Pre-Tension/1 -> sum/3  "T"
  sum/1 -> F_Mooring/1  "F_Mooring"
  Product1/1 -> sum/2  "Cm*v"
  Product/1 -> sum/1  "Km*x_cg"

== system WECSim_Lib/Constraints/Pitch/Mooring/MoorDyn ==
  Displacement : Inport
  Clock : Inport  Port=2
  Velocity : Inport  Port=3
  MoorDyn : Subsystem  InitFcn=|  StopFcn=|
      InitFcn=|
      | % Initialize MoorDyn Lib (Windows:dll or OSX:dylib)
      | if ismac
      |     loadlibrary('Lines.dylib','MoorDyn.h');
      | else
      |    if ispc
      |       loadlibrary('Lines.dll','MoorDyn.h');
      |    else
      |       disp('Cannot run MoorDyn in this platform');
      |    end
      | end
      | calllib('Lines','LinesInit',constraint.loc,[0 0 0 0 0 0]);
      StopFcn=|
      | calllib('Lines','LinesClose');
      | unloadlibrary Lines;
      settings: CloseFcn=|
      | calllib('Lines','LinesClose');
      | unloadlibrary Lines;
  F_Mooring : Outport
  wires:
  MoorDyn/1(Flines) -> F_Mooring/1
  Clock/1 -> MoorDyn/2(Clock)
  Displacement/1 -> MoorDyn/3(Displacement)
  Velocity/1 -> MoorDyn/1(Velocity)

== system WECSim_Lib/Constraints/Pitch/Mooring/Mooring Matrix ==
  note: Calculates the Mooring Force
      |
      | Mooring force = Kmooring matrix * displacement vector (relative to cg)
      | 	+ Cmooring matrix * velocity vector
      | 	- PreTension vector
      | F_Mooring = x_cg * Km  +  v * Cm  -  T
  Displacement : Inport
  Velocity : Inport  Port=2
  Center of Gravity2 : Constant  Value=constraint.mooring.c
  Mooring K Matrix : Constant  Value=constraint.mooring.k
  Mooring Pre-Tension : Constant  Value=constraint.mooring.preTension
  Product : Product  Multiplication=Matrix(*)
  Product1 : Product  Multiplication=Matrix(*)
  sum : Sum  Inputs=--+
  F_Mooring : Outport
  wires:
  Center of Gravity2/1 -> Product1/1  "Cm"
  Velocity/1 -> Product1/2  "v"
  Mooring K Matrix/1 -> Product/1  "Km"
  Displacement/1 -> Product/2  "x"
  Mooring Pre-Tension/1 -> sum/3  "T"
  sum/1 -> F_Mooring/1  "F_Mooring"
  Product1/1 -> sum/2  "Cm*v"
  Product/1 -> sum/1  "Km*x_cg"

== system WECSim_Lib/Constraints/Surge/Mooring/MoorDyn ==
  Displacement : Inport
  Clock : Inport  Port=2
  Velocity : Inport  Port=3
  MoorDyn : Subsystem  InitFcn=|  StopFcn=|
      InitFcn=|
      | % Initialize MoorDyn Lib (Windows:dll or OSX:dylib)
      | if ismac
      |     loadlibrary('Lines.dylib','MoorDyn.h');
      | else
      |    if ispc
      |       loadlibrary('Lines.dll','MoorDyn.h');
      |    else
      |       disp('Cannot run MoorDyn in this platform');
      |    end
      | end
      | calllib('Lines','LinesInit',constraint.loc,[0 0 0 0 0 0]);
      StopFcn=|
      | calllib('Lines','LinesClose');
      | unloadlibrary Lines;
      settings: CloseFcn=|
      | calllib('Lines','LinesClose');
      | unloadlibrary Lines;
  F_Mooring : Outport
  wires:
  MoorDyn/1(Flines) -> F_Mooring/1
  Clock/1 -> MoorDyn/2(Clock)
  Displacement/1 -> MoorDyn/3(Displacement)
  Velocity/1 -> MoorDyn/1(Velocity)

== system WECSim_Lib/Constraints/Surge/Mooring/Mooring Matrix ==
  note: Calculates the Mooring Force
      |
      | Mooring force = Kmooring matrix * displacement vector (relative to cg)
      | 	+ Cmooring matrix * velocity vector
      | 	- PreTension vector
      | F_Mooring = x_cg * Km  +  v * Cm  -  T
  Displacement : Inport
  Velocity : Inport  Port=2
  Center of Gravity2 : Constant  Value=constraint.mooring.c
  Mooring K Matrix : Constant  Value=constraint.mooring.k
  Mooring Pre-Tension : Constant  Value=constraint.mooring.preTension
  Product : Product  Multiplication=Matrix(*)
  Product1 : Product  Multiplication=Matrix(*)
  sum : Sum  Inputs=--+
  F_Mooring : Outport
  wires:
  Center of Gravity2/1 -> Product1/1  "Cm"
  Velocity/1 -> Product1/2  "v"
  Mooring K Matrix/1 -> Product/1  "Km"
  Displacement/1 -> Product/2  "x"
  Mooring Pre-Tension/1 -> sum/3  "T"
  sum/1 -> F_Mooring/1  "F_Mooring"
  Product1/1 -> sum/2  "Cm*v"
  Product/1 -> sum/1  "Km*x_cg"

== system WECSim_Lib/Body Elements/Rigid Body/B2B Subsystem/B2B/CrossCoupling ==
  note: CrossCoupling block is updated by its mask initialization, which is only called on when a simulation is run. 'From' blocks are automatically created and connected based on the number of bodies in the simulation.
  BC1 : BusCreator  Inputs=1
  BC2 : BusCreator  Inputs=1
  vel : Outport
  acc : Outport  Port=2
  wires:
  [vel1] -> BC1/1
  [acc1] -> BC2/1
  BC1/1 -> vel/1
  BC2/1 -> acc/1

== system WECSim_Lib/Body Elements/Rigid Body/Hydrostatic Restoring Force Calculation/Linear and Nonlinear Restoring Force Variant Subsystem/Linear Hydrostatic Restoring Force  ==
  note: Calculates the net buoyancy and linear restoring forces
      | 	Net Buoyancy Force in z-direction = gravity force - buoyancy force = m*g - rho*g*Vol
      | 	Linear Restoring Force = linear restoring coefficient matrix * displacement about cg vector = k * x_cg
      |
      | For a floating body, the net boyancy force = 0.
  In1 : Inport
  Add1 : Sum  Inputs=+-
  Add2 : Sum
  Assignment (Add Net Bouyancy Force to Z-Direction) : Assignment  Indices=3
  Body Mass : Constant  Value=body.hydroForce.storage.mass
  Constant1 : Constant  Value=[0 0 0 0 0 0]
  Gravity : Constant  Value=simu.g
  Linear Restioring Coefficient Matrix : Constant  Value=body.hydroForce.linearHydroRestCoef
  Product : Product
  Product1 : Product  Inputs=3
  Product2 : Product  Multiplication=Matrix(*)
  Volume : Constant  Value=body.hydroData.properties.disp_vol
  Water Density : Constant  Value=simu.rho
  Out1 : Outport
  wires:
  In1/1 -> Product2/2  "x"
  Body Mass/1 -> Product/2  "m"
  Constant1/1 -> Assignment (Add Net Bouyancy Force to Z-Direction)/1
  Assignment (Add Net Bouyancy Force to Z-Direction)/1 -> Add2/1  "Net Buoyancy Force"
  Add2/1 -> Out1/1  "F_Restoring"
  Volume/1 -> Product1/3  "Vol"
  Gravity/1 -> Product1/2, Product/1  "g"
  Water Density/1 -> Product1/1  "rho"
  Product/1 -> Add1/1  "F_Gravity"
  Product1/1 -> Add1/2  "F_Buoyancy"
  Add1/1 -> Assignment (Add Net Bouyancy Force to Z-Direction)/2
  Product2/1 -> Add2/2  "Linear Restoring Force"
  Linear Restioring Coefficient Matrix/1 -> Product2/1  "K"

== system WECSim_Lib/Body Elements/Rigid Body/Hydrostatic Restoring Force Calculation/Linear and Nonlinear Restoring Force Variant Subsystem/Nonlinear Hydrostatic Restoring Force ==
  In1 : Inport
  In2 : Inport  Port=2
  In3 : Inport  Port=3
  Add3 : Sum  Inputs=-+
  Assignment (Add Net Bouyancy Force to Z-Direction)2 : Assignment  Indices=3
  Body Mass1 : Constant  Value=body.hydroForce.storage.mass
  Center of Gravity : Constant  Value=body.hydroData.properties.cg
  Constant2 : Constant  Value=[0 0 0 0 0 0]
  Diffarction and Excitation Forces1 : MATLAB Function  TreatAsAtomicUnit=on
  Gravity2 : Constant  Value=simu.g
  Product3 : Product
  SImulation Step Time : Constant  Value=simu.dt
  STL areas : Constant  Value=body.bodyGeometry.area
  STL centers : Constant  Value=body.bodyGeometry.center
  STL normal vectors : Constant  Value=body.bodyGeometry.norm
  Simulation Fe Calc Step Time : Constant  Value=simu.dtFeNonlin
  To Workspace1 : ToWorkspace  VariableName=body1_hspressure_out  SaveFormat=Structure With Time  SampleTime=-1
      settings: Decimation=round(simu.dtOut/simu.dt,0)
  Water Density1 : Constant  Value=simu.rho
  Out1 : Outport
  wires:
  In1/1 -> Diffarction and Excitation Forces1/1(x)
  Center of Gravity/1 -> Diffarction and Excitation Forces1/8(cg)
  Assignment (Add Net Bouyancy Force to Z-Direction)2/1 -> Add3/2
  Add3/1 -> Out1/1
  Diffarction and Excitation Forces1/1(f) -> Add3/1
  Product3/1 -> Assignment (Add Net Bouyancy Force to Z-Direction)2/2
  Constant2/1 -> Assignment (Add Net Bouyancy Force to Z-Direction)2/1
  Body Mass1/1 -> Product3/2
  Gravity2/1 -> Product3/1, Diffarction and Excitation Forces1/7(g)  "g"
  Water Density1/1 -> Diffarction and Excitation Forces1/6(rho)
  STL normal vectors/1 -> Diffarction and Excitation Forces1/4(tnorm)
  STL centers/1 -> Diffarction and Excitation Forces1/3(center)
  In2/1 -> Diffarction and Excitation Forces1/2(elv)
  Diffarction and Excitation Forces1/2(p) -> To Workspace1/1
  SImulation Step Time/1 -> Diffarction and Excitation Forces1/9(dt)
  Simulation Fe Calc Step Time/1 -> Diffarction and Excitation Forces1/10(dtFe)
  In3/1 -> Diffarction and Excitation Forces1/11(t)
  STL areas/1 -> Diffarction and Excitation Forces1/5(area)

== system WECSim_Lib/Body Elements/Rigid Body/Morrison Element and ViscousDampingForceCalculation/Morrison Element Variant Subsystem/Morrison Element Off ==
  Constant : Constant  Value=[0 0 0 0 0 0]
  Out1 : Outport
  wires:
  Constant/1 -> Out1/1

== system WECSim_Lib/Body Elements/Rigid Body/Morrison Element and ViscousDampingForceCalculation/Morrison Element Variant Subsystem/Morrison Element On ==
  note: 1) Add Subsystem or Model blocks as valid variant choices.
      | 2) You cannot connect blocks at this level. At simulation, connectivity is automatically
      | determined, based on the active variant and port name matching.
  In1 : Inport
  In2 : Inport  Port=2
  In3 : Inport  Port=3
  Irregular Wave Excitation Force : Subsystem  VariantControl=sv_irregularWaves
  No Wave Excitation Force : Subsystem  VariantControl=sv_noWave
  Regular Wave Excitation Force : Subsystem  VariantControl=sv_regularWaves
  Out1 : Outport

== system WECSim_Lib/Body Elements/Rigid Body/Nonlinear Wave Elevation/Linear or Instantaneous Free Surface/Instantaneous Water Free Surface   ==
  In1 : Inport
  In2 : Inport  Port=2
  Center of Gravity : Constant  Value=body.hydroData.properties.cg
  Frequency Spacing : Constant  Value=waves.dw
  Instantaneous FS : MATLAB Function  TreatAsAtomicUnit=on
  Ramp Time : Constant  Value=simu.rampT
  STL Centers : Constant  Value=body.bodyGeometry.center
  Simulation Time Step : Constant  Value=simu.dt
  Time Step for Non-Linear Forces : Constant  Value=simu.dtFeNonlin
  Wave Amplitude : Constant  Value=waves.A
  Wave Direction : Constant  Value=waves.waveDir
  Wave Frequency : Constant  Value=waves.w
  Wave Number : Constant  Value=waves.k
  Wave Random Phase : Constant  Value=waves.phaseRand
  Wave Type Number : Constant  Value=waves.typeNum
  Out1 : Outport
  wires:
  Instantaneous FS/1(f) -> Out1/1
  STL Centers/1 -> Instantaneous FS/2(center)
  Center of Gravity/1 -> Instantaneous FS/3(cg)
  Wave Number/1 -> Instantaneous FS/7(k)
  Wave Frequency/1 -> Instantaneous FS/5(w)
  Wave Type Number/1 -> Instantaneous FS/8(typeNum)
  Ramp Time/1 -> Instantaneous FS/10(rampT)
  Wave Random Phase/1 -> Instantaneous FS/11(phaseRand)
  Frequency Spacing/1 -> Instantaneous FS/6(dw)
  In2/1 -> Instantaneous FS/9(t)
  In1/1 -> Instantaneous FS/1(x)
  Wave Direction/1 -> Instantaneous FS/12(waveDir)
  Simulation Time Step/1 -> Instantaneous FS/13(dt)
  Time Step for Non-Linear Forces/1 -> Instantaneous FS/14(dtFe)
  Wave Amplitude/1 -> Instantaneous FS/4(AH)

== system WECSim_Lib/Body Elements/Rigid Body/Nonlinear Wave Elevation/Linear or Instantaneous Free Surface/Mean Water Free Surface  ==
  zero : Constant  Value=0
  Out1 : Outport
  wires:
  zero/1 -> Out1/1
